simulink model "Vehicle_Dynamics_Testrig_org"  (Simulink 10.0)
settings: Solver=ode23t  StartTime=0.0  StopTime=400  RelTol=1e-3  AbsTol=1e-4  EnableMultiTasking=on
PostLoadFcn:
  | warning off Simulink:Engine:SaveWithDisabledLinks_Warning
  | warning off Simulink:Engine:UsingDefaultMaxStepSize
undefined symbols (not defined in the file): sigbuilder_block
libraries: fl_lib x12, nesl_utility x7, sdl_lib x4, DCT_Vehicle_Dynamics_Lib x1
Description:
  | Copyright 2014-2017 The MathWorks, Inc.
settings Model: Creator=smiller  LastModifiedBy=bhisma
settings SolverCC: AutoScaleAbsTol=off
settings DataIOCC: LimitDataPoints=on  SignalLoggingSaveFormat=ModelDataLogs
settings OptimizationCC: ExpressionDepthLimit=2147483647
settings DebuggingCC: SolverPrmCheckMsg=warning  FcnCallInpInsideContextMsg=warning  AllowSymbolicDim=off  StateNameClashWarn=warning
settings GRTTargetCC: GeneratePreprocessorConditionals=Disable all
settings ConfigComp: CovExternalEMLEnable=off  CovSFcnEnable=off
settings SimscapeCC: SimscapeNormalizeSystem=off  SimscapeNominalValues="[{\"value\":\"10\",\"unit\":\"V\"},{\"value\":\"1\",\"unit\":\"A\"},{\"value\":\"10\",\"unit\":\"N*m\"},{\"value\":\"10\",\"unit\":\"bar\"},{\"value\":\"100\",\"unit\":\"kJ/kg\"},{\"value\":\"1\",\"unit\":\"kW\"},{\"value\":\"300\",\"unit\":\"K\"},{\"value\":\"100\",\"unit\":\"cm^3/s\"},{\"value\":\"1\",\"unit\":\"kN\"},{\"value\":\"1\",\"unit\":\"g/cm^3\"},{\"value\":\"1\",\"unit\":\"l\"},{\"value\":\"1\",\"unit\":\"cm^2\"},{\"value\":\"60\",\"unit\":\"Hz\"}]"

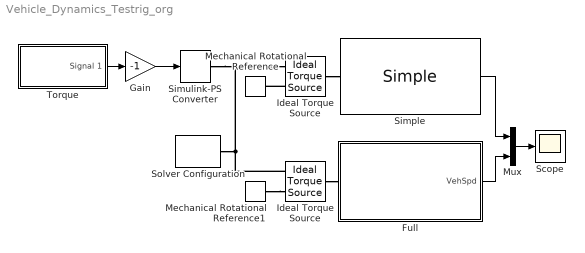
== system Vehicle_Dynamics_Testrig_org ==
  Full : Subsystem  AncestorBlock=DCT_Vehicle_Dynamics_Lib/Full
      mask Display:
      | image(imread('DCT_Vehicle_Dynamics_Full_IMAGE.jpg'));
      | port_label('LConn',1,'Sh');
      | port_label('output',1,'Spd');
  Gain : Gain  Gain=-1
  Ideal Torque Source : fl_lib/Mechanical/Mechanical Sources/Ideal Torque Source
  "Ideal Torque Source " : fl_lib/Mechanical/Mechanical Sources/Ideal Torque Source
  Mechanical Rotational Reference : fl_lib/Mechanical/Rotational Elements/Mechanical Rotational Reference
  Mechanical Rotational Reference1 : fl_lib/Mechanical/Rotational Elements/Mechanical Rotational Reference
  Mux : Mux  Inputs=2
  Scope : Scope
  Simple : DCT_Vehicle_Dynamics_Lib/Simple  mass=DCT_Param.Vehicle.Mass  area=DCT_Param.Vehicle.Frontal_Area  Cd=DCT_Param.Vehicle.Aero_Drag_Coeff  radius=DCT_Param.Vehicle.Tire.Radius  wheel_inertia=DCT_Param.Vehicle.Tire.Inertia  gear_ratio=DCT_Param.Vehicle.Final_Drive_Ratio
  Simulink-PS Converter : nesl_utility/Simulink-PS Converter  PhysicalDomain=network_engine_domain  SubClassName=ps_input  LeftPortType=input  RightPortType=output  PseudoPeriodic=off  Frequencies=[]  NoiseDistribution=none  NoiseParameters=[]  Unit=1  AffineConversion=off  FilteringAndDerivatives=zero  SimscapeFilterOrder=1  InputFilterTimeConstant=.001  UdotUserProvided=0
  Solver Configuration : nesl_utility/Solver Configuration  PhysicalDomain=network_engine_domain  SubClassName=solver  LeftPortType=input  RightPortType=generic  Tones=[]  Harmonics=[]  SimulateNoise=off  Profile=off  UseLocalSampling=off  EnableSwitchedLinearOptims=on  FrequencyDomain=off  UseCCode=off  RelTol=0.001  AbsTol=1e-06  MinStep=1e-09  ToWorkspace=off  RevertToSquareIcSolve=off  NumHomotopyIterations=100  PhasorMode=off  PhasorModeNumHarmonics=1  DoDC=off  ResidualTolerance=1e-9  UseLocalSolver=off  LocalSolverChoice=NE_BACKWARD_EULER_ADVANCER  LocalSolverSampleTime=.001  DoFixedCost=off  MaxNonlinIter=3  MaxModeIter=2  LinearAlgebra=Sparse  EquationFormulation=NE_TIME_EF  DelaysMemoryBudget=1024  AutomaticFiltering=on  FilteringTimeConstant=0.001  PartitionStorageMethod=AS_NEEDED  PartitionMemoryBudget=1024  PartitionMethod=FAST
  Torque : Subsystem  Tag=STV Subsys  LoadFcn=sigbuilder_block('load');  StartFcn=sigbuilder_block('start');  StopFcn=sigbuilder_block('stop');  ClipboardFcn=sigbuilder_block('clipboard');  mask(Sigbuilder block){tuvar=[0:10]}
      mask help: Create and generate interchangeable groups of signals whose waveforms are piecewise linear.
      mask init:
      | if ~strcmp(get_param(bdroot(gcbh),'SimulationStatus'),'stopped') tuvar = sigbuilder_block('maskInit'); end
      settings: CopyFcn=sigbuilder_block('copy');  DeleteFcn=sigbuilder_block('delete');  ModelCloseFcn=sigbuilder_block('modelClose');  PreSaveFcn=sigbuilder_block('preSave');  PauseFcn=sigbuilder_block('pause')  ContinueFcn=sigbuilder_block('continue')  NameChangeFcn=sigbuilder_block('namechange');  OpenFcn=sigbuilder_block('open',[437.25 199.5 550.5 399.75 ]);  CloseFcn=sigbuilder_block('close');
      mask Display: plot(0, 0, 100, 100,[2, 2, 32, 32, 2], [68, 8, 8, 68, 68],[32, 2], [38, 38], [32, 19, 2],[53, 60, 44], [32, 17, 17, 2],[16, 16, 31, 31]);txt = getActiveGroup(gcbh);text(2, 100, txt,'verticalAlignment', 'top');
  wires:
  Simple/1 -> Mux/1
  Mux/1 -> Scope/1
  Full/1(VehSpd) -> Mux/2
  Torque/1(Signal 1) -> Gain/1
  Gain/1 -> Simulink-PS Converter/1
  connections:
  Ideal Torque Source/LConn1 -- Simple/LConn1
  Ideal Torque Source/RConn2 -- Mechanical Rotational Reference/LConn1
  "Ideal Torque Source "/RConn1 -- Ideal Torque Source/RConn1 -- Simulink-PS Converter/RConn1 -- Solver Configuration/RConn1
  Mechanical Rotational Reference1/LConn1 -- "Ideal Torque Source "/RConn2
  "Ideal Torque Source "/LConn1 -- Full/LConn1

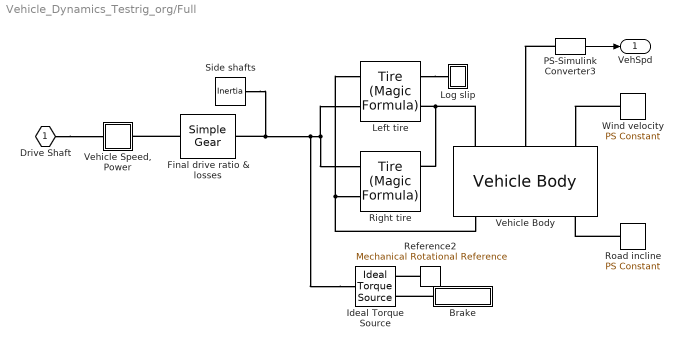
== system Vehicle_Dynamics_Testrig_org/Full ==
  Brake : Subsystem
  Final drive ratio & losses : sdl_lib/Gears/Simple Gear  ratio=DCT_Param.Vehicle.Final_Drive_Ratio  rotation_direction=2  friction_model=1  T_noload=0.1 N*m  T_nom=5 N*m  efficiency_nom=0.8  efficiency=DCT_Param.Vehicle.Final_Drive_Efficiency  mu_visc=[0 0] N*m/(rad/s)  w_thr=DCT_Param.Vehicle.Final_Drive_Vel_Thresh rad/s  pwr_thr=0.001 W  enable_faults=simscape.enum.onoff.off  efficiency_fault=0.05  external_fault=simscape.enum.onoff.off  temporal_fault=simscape.enum.onoff.off  fault_time=5 s  fault_angles=pi / 12 rad  report_fault=1  temperature_TLU=[ 280 300 320 ] K  load_TLU=[ 1 5 10 ] N*m  efficiency_TLU=[ 0.95 0.9 0.85 ]  efficiency_TLU2=[ 0.85 0.8 0.75; 0.95 0.9 0.85; 0.85 0.8 0.7 ]  thermal_mass=50 J/K  T_init=300 K
      settings: SourceProductName=Simscape Driveline
  Ideal Torque Source : fl_lib/Mechanical/Mechanical Sources/Ideal Torque Source
  Left tire : sdl_lib/Tires & Vehicles/Tire (Magic Formula)  parameterization=3  F_z1=3000 N  F_x1=3500 N  kappa1=10  B_m=10  C_m=1.9  D_m=1  E_m=0.97  fz0=DCT_Param.Vehicle.Tire.Nominal_Vertical_Load N  p_Cx=DCT_Param.Vehicle.Tire.C_Coeff  p_Dx=DCT_Param.Vehicle.Tire.D_Coeff  p_Ex=DCT_Param.Vehicle.Tire.E_Coeff  p_Kx=DCT_Param.Vehicle.Tire.BCD_Coeff  p_Hx=DCT_Param.Vehicle.Tire.H_Coeff  p_Vx=DCT_Param.Vehicle.Tire.V_Coeff  v_tr_thr=DCT_Param.Vehicle.Tire.Slip_Vel_Thresh m/s  r_e=DCT_Param.Vehicle.Tire.Radius m  model_compliance=0  stiffness=1e+6 N/m  damping=1000 N/(m/s)  model_inertia=1  inertia=DCT_Param.Vehicle.Tire.Inertia kg*m^2  initial_velocity=DCT_Param.Vehicle.Tire.Initial_Velocity rpm  model_resistance=0  resistance_model=1  coeff=0.015  p_tire=250e3 Pa  alpha=-0.003  beta=0.97  coeff_a=84e-4  coeff_b=6.2e-4 s/m  coeff_c=1.6e-4 s^2/m^2  v_thr=1e-3 m/s
      settings: SourceProductName=Simscape Driveline
  Log slip : Subsystem
  PS-Simulink Converter3 : nesl_utility/PS-Simulink Converter  PhysicalDomain=network_engine_domain  SubClassName=ps_output  LeftPortType=input  RightPortType=output  PseudoPeriodic=off  Frequencies=[]  Unit=km/hr  AffineConversion=off
  Reference2 : fl_lib/Mechanical/Rotational Elements/Mechanical Rotational Reference
  Right tire : sdl_lib/Tires & Vehicles/Tire (Magic Formula)  parameterization=3  F_z1=3000 N  F_x1=3500 N  kappa1=10  B_m=10  C_m=1.9  D_m=1  E_m=0.97  fz0=DCT_Param.Vehicle.Tire.Nominal_Vertical_Load N  p_Cx=DCT_Param.Vehicle.Tire.C_Coeff  p_Dx=DCT_Param.Vehicle.Tire.D_Coeff  p_Ex=DCT_Param.Vehicle.Tire.E_Coeff  p_Kx=DCT_Param.Vehicle.Tire.BCD_Coeff  p_Hx=DCT_Param.Vehicle.Tire.H_Coeff  p_Vx=DCT_Param.Vehicle.Tire.V_Coeff  v_tr_thr=DCT_Param.Vehicle.Tire.Slip_Vel_Thresh m/s  r_e=DCT_Param.Vehicle.Tire.Radius m  model_compliance=0  stiffness=1e+6 N/m  damping=1000 N/(m/s)  model_inertia=1  inertia=DCT_Param.Vehicle.Tire.Inertia kg*m^2  initial_velocity=DCT_Param.Vehicle.Tire.Initial_Velocity rpm  model_resistance=0  resistance_model=1  coeff=0.015  p_tire=250e3 Pa  alpha=-0.003  beta=0.97  coeff_a=84e-4  coeff_b=6.2e-4 s/m  coeff_c=1.6e-4 s^2/m^2  v_thr=1e-3 m/s
      settings: SourceProductName=Simscape Driveline
  Road incline : fl_lib/Physical Signals/Sources/PS Constant  constant=0
  Side shafts : fl_lib/Mechanical/Rotational Elements/Inertia  inertia=DCT_Param.Vehicle.Side_Shaft_Inertia kg*m^2  w_specify=on  w_priority=High  w=DCT_Param.Vehicle.Side_Shaft_Initial_Velocity rad/s  w_nominal_specify=off  w_nominal_unit=rad/s  w_nominal_value=1  t_specify=off  t_priority=High  t=0 N*m  t_nominal_specify=off  t_nominal_unit=N*m  t_nominal_value=1
  Vehicle Body : sdl_lib/Tires & Vehicles/Vehicle Body  mass=DCT_Param.Vehicle.Mass kg  n_w=DCT_Param.Vehicle.Wheels_Per_Axle  x_f=DCT_Param.Vehicle.Distance_CG_FrontAxle m  x_r=DCT_Param.Vehicle.Distance_CG_RearAxle m  y_c=DCT_Param.Vehicle.Distance_CG_Ground m  mass_var=simscape.enum.onoff.off  model_pitch=simscape.enum.onoff.off  inertia=4000 kg*m^2  suspension_model=sdl.enum.linearTLU.linear  k_f=1e4 N/m  b_f=1e4 N/(m/s)  k_r=1e4 N/m  b_r=1e4 N/(m/s)  k_f_TLU=[-2000, -1000, 0, 1000, 2000] N  x_f_TLU=[-.4, -.2, 0, .2, .4] m  b_f_TLU=[-200, -100, 0, 100, 200] N  v_f_TLU=[-4, -2, 0, 2, 4] m/s  k_r_TLU=[-2000, -1000, 0, 1000, 2000] N  x_r_TLU=[-.4, -.2, 0, .2, .4] m  b_r_TLU=[-200, -100, 0, 100, 200] N  v_r_TLU=[-4, -2, 0, 2, 4] m/s  interp_method=simscape.enum.interpolation.linear  extrap_method=simscape.enum.extrapolation.linear  model_hardstop=simscape.enum.onoff.off  upper_bound_f=.25 m  lower_bound_f=-.25 m  stop_k_f=1e6 N/m  stop_b_f=150 N/(m/s)  upper_bound_r=.25 m  lower_bound_r=-.25 m  stop_k_r=1e6 N/m  stop_b_r=150 N/(m/s)  initial_pitch=0 rad  initial_pitch_rate=0 rad/s  g=9.81 m/s^2  liftoff_warning=simscape.enum.onoff.off  area=DCT_Param.Vehicle.Frontal_Area m^2  Cd=DCT_Param.Vehicle.Aero_Drag_Coeff  rho=1.18 kg/m^3  v_specify=on  v_priority=High  v=DCT_Param.Vehicle.Initial_Velocity m/s  v_nominal_specify=off  v_nominal_unit=m/s  v_nominal_value=1
      settings: SourceProductName=Simscape Driveline
  "Vehicle Speed, Power" : Subsystem
      mask Display: disp('S')
  Wind velocity : fl_lib/Physical Signals/Sources/PS Constant  constant=0
  Drive Shaft : PMIOPort  Side=Left
  VehSpd : Outport
  wires:
  PS-Simulink Converter3/1 -> VehSpd/1
  connections:
  Ideal Torque Source/LConn1 -- Final drive ratio & losses/RConn1 -- Side shafts/LConn1 -- Left tire/LConn2 -- Right tire/LConn2
  Final drive ratio & losses/LConn1 -- "Vehicle Speed, Power"/RConn1
  Reference2/LConn1 -- Ideal Torque Source/RConn2
  Brake/RConn1 -- Ideal Torque Source/RConn1
  Drive Shaft/RConn1 -- "Vehicle Speed, Power"/LConn1
  Left tire/RConn1 -- Log slip/LConn1
  PS-Simulink Converter3/LConn1 -- Vehicle Body/LConn2
  Wind velocity/RConn1 -- Vehicle Body/LConn3
  Road incline/RConn1 -- Vehicle Body/RConn3
  Vehicle Body/RConn1 -- Left tire/LConn1 -- Right tire/LConn1
  Vehicle Body/LConn1 -- Left tire/RConn2 -- Right tire/RConn2

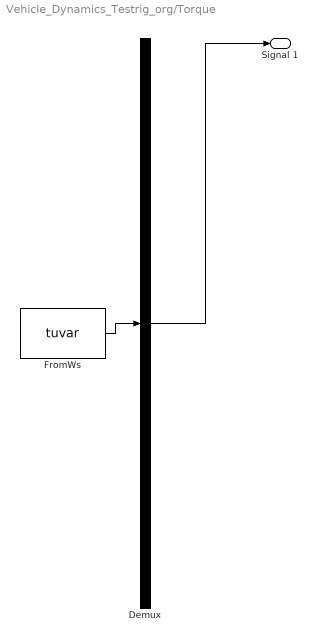
== system Vehicle_Dynamics_Testrig_org/Torque ==
  Demux : Demux  Tag=STV Demux  Outputs=1
  FromWs : FromWorkspace  Tag=STV FromWs  VariableName=tuvar  SampleTime=0  SigBuilderData=DataTag0  VnvData=DataTag1
      SigBuilderData=|
      | common.afterFinalStr = 'Extrapolate'
      | common.sampleTime = 0
      | dataSet.timeRange = [0 400]
      | dataSet.name = 'Group 1'
      | sbobj.Groups.Name = 'Group 1'
      | sbobj.Groups.Signals.Name = 'Signal 1'
      | sbobj.Groups.Signals.XData = [0 6 6 50 50 150 150 170 170 400]
      | sbobj.Groups.Signals.YData = [0 0 100 100 0 0 100 100 0 0]
      | sbobj.Groups.TimeRange = [0 400]
  Signal 1 : Outport  Tag=STV Outport
  wires:
  Demux/1 -> Signal 1/1
  FromWs/1 -> Demux/1

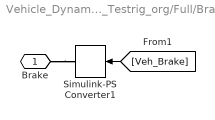
== system Vehicle_Dynamics_Testrig_org/Full/Brake ==
  Simulink-PS Converter1 : nesl_utility/Simulink-PS Converter  PhysicalDomain=network_engine_domain  SubClassName=ps_input  LeftPortType=input  RightPortType=output  PseudoPeriodic=off  Frequencies=[]  NoiseDistribution=none  NoiseParameters=[]  Unit=1  AffineConversion=off  FilteringAndDerivatives=zero  SimscapeFilterOrder=1  InputFilterTimeConstant=.001  UdotUserProvided=0
  Brake : PMIOPort  Side=Right
  wires:
  [Veh_Brake] -> Simulink-PS Converter1/1
  connections:
  Brake/RConn1 -- Simulink-PS Converter1/RConn1

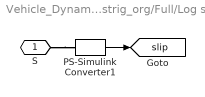
== system Vehicle_Dynamics_Testrig_org/Full/Log slip ==
  PS-Simulink Converter1 : nesl_utility/PS-Simulink Converter  PhysicalDomain=network_engine_domain  SubClassName=ps_output  LeftPortType=input  RightPortType=output  PseudoPeriodic=off  Frequencies=[]  Unit=1  AffineConversion=off
  S : PMIOPort  Side=Left
  tag scope: slip=global
  wires:
  PS-Simulink Converter1/1 -> [slip]
  connections:
  S/RConn1 -- PS-Simulink Converter1/LConn1

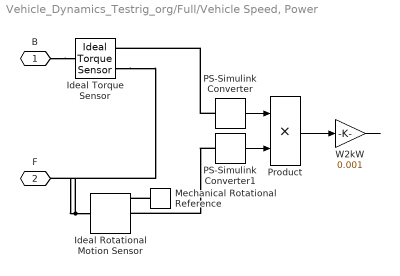
== system Vehicle_Dynamics_Testrig_org/Full/Vehicle Speed, Power ==
  Ideal Rotational Motion Sensor : fl_lib/Mechanical/Mechanical Sensors/Ideal Rotational Motion Sensor  offset=0 rad
  Ideal Torque Sensor : fl_lib/Mechanical/Mechanical Sensors/Ideal Torque Sensor
  Mechanical Rotational Reference : fl_lib/Mechanical/Rotational Elements/Mechanical Rotational Reference
  PS-Simulink Converter : nesl_utility/PS-Simulink Converter  PhysicalDomain=network_engine_domain  SubClassName=ps_output  LeftPortType=input  RightPortType=output  PseudoPeriodic=off  Frequencies=[]  Unit=N*m  AffineConversion=off
  PS-Simulink Converter1 : nesl_utility/PS-Simulink Converter  PhysicalDomain=network_engine_domain  SubClassName=ps_output  LeftPortType=input  RightPortType=output  PseudoPeriodic=off  Frequencies=[]  Unit=rad/s  AffineConversion=off
  Product : Product  RndMeth=Zero
  W2kW : Gain  Gain=0.001
  B : PMIOPort  Side=Left
  F : PMIOPort  Port=2  Side=Right
  wires:
  W2kW/1 -> ?
  Product/1 -> W2kW/1
  PS-Simulink Converter/1 -> Product/1
  PS-Simulink Converter1/1 -> Product/2
  connections:
  Mechanical Rotational Reference/LConn1 -- Ideal Rotational Motion Sensor/RConn1
  Ideal Rotational Motion Sensor/LConn1 -- F/RConn1 -- Ideal Torque Sensor/RConn1
  B/RConn1 -- Ideal Torque Sensor/LConn1
  PS-Simulink Converter/LConn1 -- Ideal Torque Sensor/RConn2
  PS-Simulink Converter1/LConn1 -- Ideal Rotational Motion Sensor/RConn2
